simulink model "gyroYawLoop"  (R2015a)
settings: Solver=ode45  StartTime=0.0  StopTime=20  RelTol=1e-3
values from neighbouring files (symbols this model uses):
  dt = 0.02    [startup.m]
  innerIntegralGain = 0.05    [startup.m]
  innerProportionalGain = 1    [startup.m]
  outerIntegralGain = 0    [startup.m]
  outerProportionalGain = 4    [startup.m]
  plantGain = 12    [startup.m]
  plantTorqueOffset = 0.2    [startup.m]
  torqueOffset = 0    [startup.m]
libraries: simulink x2, vrlib x1
settings Model: Creator=johnz  LastModifiedBy=johnz
settings DataIOCC: SaveOutput=off  SaveTime=off  OutputSaveName=totalAngularError

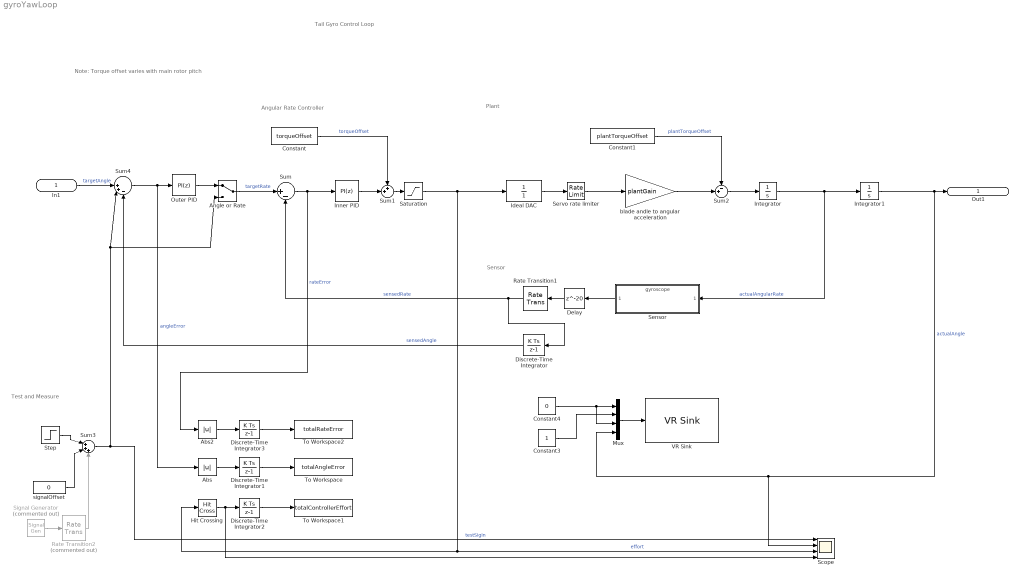
== system gyroYawLoop ==
  note: Angular Rate Controller
  note: Sensor
  note: Test and Measure
  note: Tail Gyro Control Loop
  note: Note: Torque offset varies with main rotor pitch
  note: Plant
  In1 : Inport  SampleTime=dt
  Abs : Abs
  Abs2 : Abs
  Angle or Rate : ManualSwitch
  Constant : Constant  Value=torqueOffset  SampleTime=dt
  Constant1 : Constant  Value=plantTorqueOffset
  Constant3 : Constant
  Constant4 : Constant  Value=0
  Delay : Delay  DelayLength=20
  Discrete-Time Integrator{,1..3} (4 alike) : DiscreteIntegrator  InitialConditionSetting=State (most efficient)  SampleTime=-1
  Hit Crossing : HitCross  HitCrossingOffset=0.1
  Ideal DAC : TransferFcn  Denominator=[1]
  Inner PID : simulink/Continuous/PID Controller  Controller=PI  TimeDomain=Discrete-time  SampleTime=dt  IntegratorMethod=Forward Euler  FilterMethod=Forward Euler  Form=Parallel  UseFilter=on  ControllerParametersSource=internal  P=innerProportionalGain  I=innerIntegralGain  D=0  N=100  InitialConditionSource=internal  InitialConditionForIntegrator=0  InitialConditionForFilter=0  ExternalReset=none  LimitOutput=off  UpperSaturationLimit=inf  LowerSaturationLimit=-inf  LinearizeAsGain=off  AntiWindupMode=none  Kb=1  TrackingMode=off  Kt=1  PParamMin=[]  PParamMax=[]  IParamMin=[]  IParamMax=[]  DParamMin=[]  DParamMax=[]  NParamMin=[]  NParamMax=[]  KbParamMin=[]  KbParamMax=[]  KtParamMin=[]  KtParamMax=[]  POutMin=[]  POutMax=[]  IOutMin=[]  IOutMax=[]  DOutMin=[]  DOutMax=[]  NOutMin=[]  NOutMax=[]  KbOutMin=[]  KbOutMax=[]  KtOutMin=[]  KtOutMax=[]  IntegratorOutMin=[]  IntegratorOutMax=[]  FilterOutMin=[]  FilterOutMax=[]  SumOutMin=[]  SumOutMax=[]  SumI1OutMin=[]  SumI1OutMax=[]  SumI2OutMin=[]  SumI2OutMax=[]  SumI3OutMin=[]  SumI3OutMax=[]  SumDOutMin=[]  SumDOutMax=[]  SaturationOutMin=[]  SaturationOutMax=[]  IntegratorContinuousStateAttributes=''  IntegratorStateMustResolveToSignalObject=off  IntegratorRTWStateStorageClass=Auto  FilterContinuousStateAttributes=''  FilterStateMustResolveToSignalObject=off  FilterRTWStateStorageClass=Auto  DifferentiatorICPrevScaledInput=0  DifferentiatorOutMin=[]  DifferentiatorOutMax=[]
  Integrator : Integrator
  Integrator1 : Integrator
  Mux : Mux
  Outer PID : simulink/Continuous/PID Controller  Controller=PI  TimeDomain=Discrete-time  SampleTime=dt  IntegratorMethod=Forward Euler  FilterMethod=Forward Euler  Form=Parallel  UseFilter=on  ControllerParametersSource=internal  P=outerProportionalGain  I=outerIntegralGain  D=0.02  N=100  InitialConditionSource=internal  InitialConditionForIntegrator=0  InitialConditionForFilter=0  ExternalReset=none  LimitOutput=off  UpperSaturationLimit=inf  LowerSaturationLimit=-inf  LinearizeAsGain=off  AntiWindupMode=none  Kb=1  TrackingMode=off  Kt=1  PParamMin=[]  PParamMax=[]  IParamMin=[]  IParamMax=[]  DParamMin=[]  DParamMax=[]  NParamMin=[]  NParamMax=[]  KbParamMin=[]  KbParamMax=[]  KtParamMin=[]  KtParamMax=[]  POutMin=[]  POutMax=[]  IOutMin=[]  IOutMax=[]  DOutMin=[]  DOutMax=[]  NOutMin=[]  NOutMax=[]  KbOutMin=[]  KbOutMax=[]  KtOutMin=[]  KtOutMax=[]  IntegratorOutMin=[]  IntegratorOutMax=[]  FilterOutMin=[]  FilterOutMax=[]  SumOutMin=[]  SumOutMax=[]  SumI1OutMin=[]  SumI1OutMax=[]  SumI2OutMin=[]  SumI2OutMax=[]  SumI3OutMin=[]  SumI3OutMax=[]  SumDOutMin=[]  SumDOutMax=[]  SaturationOutMin=[]  SaturationOutMax=[]  IntegratorContinuousStateAttributes=''  IntegratorStateMustResolveToSignalObject=off  IntegratorRTWStateStorageClass=Auto  FilterContinuousStateAttributes=''  FilterStateMustResolveToSignalObject=off  FilterRTWStateStorageClass=Auto  DifferentiatorICPrevScaledInput=0  DifferentiatorOutMin=[]  DifferentiatorOutMax=[]
  Rate Transition1 : RateTransition  OutPortSampleTime=dt
  Rate Transition2 : RateTransition  Commented=on  OutPortSampleTime=dt
  Saturation : Saturate  UpperLimit=1  LowerLimit=-1
  Scope : Scope  NumInputPorts=4
      settings: TickLabels=on  TimeRange=3  YMin=0~-0.05~-0.05~-5  YMax=1~1.05~1~5
  Sensor : ModelReference  ModelNameDialog=gyroscope.slx  ParameterArgumentNames=randomSeed  ParameterArgumentValues=1  SimulationMode=Normal  ModelReferenceVersion=1.23  CopyOfModelName=gyroscope.slx  DefaultDataLogging=on
  Servo rate limiter : RateLimiter  RisingSlewLimit=15  FallingSlewLimit=-15  SampleTimeMode=inherited
  Signal Generator : SignalGenerator  Commented=on  WaveForm=square  Amplitude=0.5  VectorParams1D=off
  Step : Step  SampleTime=dt
  Sum : Sum  Inputs=|+-
  Sum1 : Sum  Inputs=++|
  Sum2 : Sum  Inputs=-+|
  Sum3 : Sum  Inputs=|+++
  Sum4 : Sum  Inputs=||++-
  To Workspace : ToWorkspace  VariableName=totalAngleError  SampleTime=-1
      settings: MaxDataPoints=1
  To Workspace1 : ToWorkspace  VariableName=totalControllerEffort  SampleTime=-1
      settings: MaxDataPoints=1
  To Workspace2 : ToWorkspace  VariableName=totalRateError  SampleTime=-1
      settings: MaxDataPoints=1
  VR Sink : vrlib/VR Sink  InstantiateOnLoad=on  SampleTime=.001  ViewEnable=on  RemoteChange=off  RemoteView=off  FieldsWritten=Helicopter.rotation.4.1.1.double  WorldFileName=animation\animation_world.wrl  AutoView=off  VideoDimensions=[]  AllowVariableSize=off
  blade andle to angular acceleration : Gain  Gain=plantGain
  signalOffset : Constant  Value=0  SampleTime=dt
  Out1 : Outport
  wires:
  Sum4/1 -> Outer PID/1, Abs/1  "angleError"
  Constant/1 -> Sum1/1  "torqueOffset"
  Sum/1 -> Inner PID/1, Abs2/1  "rateError"
  Sum1/1 -> Saturation/1
  Ideal DAC/1 -> Servo rate limiter/1
  Integrator/1 -> Integrator1/1, Sensor/1  "actualAngularRate"
  Constant4/1 -> Mux/3, Mux/1
  Mux/1 -> VR Sink/1
  Constant3/1 -> Mux/2
  Inner PID/1 -> Sum1/2
  Sensor/1 -> Delay/1
  signalOffset/1 -> Sum3/2
  In1/1 -> Sum4/1  "targetAngle"
  Sum3/1 -> Scope/1, Angle or Rate/2, Sum4/2  "testSigIn"
  Integrator1/1 -> Out1/1, Scope/2, Mux/4  "actualAngle"
  Discrete-Time Integrator/1 -> Sum4/3  "sensedAngle"
  Servo rate limiter/1 -> blade andle to angular acceleration/1
  blade andle to angular acceleration/1 -> Sum2/2
  Sum2/1 -> Integrator/1
  Constant1/1 -> Sum2/1  "plantTorqueOffset"
  Step/1 -> Sum3/1
  Discrete-Time Integrator1/1 -> To Workspace/1
  Delay/1 -> Rate Transition1/1
  Rate Transition1/1 -> Sum/2, Discrete-Time Integrator/1  "sensedRate"
  Abs/1 -> Discrete-Time Integrator1/1
  Saturation/1 -> Hit Crossing/1, Scope/3, Ideal DAC/1  "effort"
  Hit Crossing/1 -> Scope/4, Discrete-Time Integrator2/1
  Signal Generator/1 -> Rate Transition2/1
  Rate Transition2/1 -> Sum3/3
  Outer PID/1 -> Angle or Rate/1
  Angle or Rate/1 -> Sum/1  "targetRate"
  Discrete-Time Integrator3/1 -> To Workspace2/1
  Abs2/1 -> Discrete-Time Integrator3/1
  Discrete-Time Integrator2/1 -> To Workspace1/1
